simulink model "Factorial_Task"  (R2018b)
settings: Solver=FixedStepDiscrete  StartTime=0.0  StopTime=10.0  RelTol=1e-3
settings Model: Creator=karim  LastModifiedBy=karim
settings OptimizationCC: DefaultParameterBehavior=Inlined  EnhancedBackFolding=on  PassReuseOutputArgsAs=Individual arguments  OptimizeBlockOrder=speed  DifferentSizesBufferReuse=on  OptimizationCustomize=off
settings DebuggingCC: UnderspecifiedInitializationDetection=Classic  MergeDetectMultiDrivingBlocksExec=none  ParameterTunabilityLossMsg=error
settings ModelReferenceCC: PropagateSignalLabelsOutOfModel=off
settings SFSimCC: MATLABDynamicMemAlloc=off
settings RTWCC: SystemTargetFile=ert.tlc  GenCodeOnly=on  TemplateMakefile=ert_default_tmf  GenerateReport=on  IncludeHyperlinkInReport=on  LaunchReport=on  GenerateTraceInfo=on  GenerateTraceReport=on  GenerateTraceReportSl=on  GenerateTraceReportSf=on  GenerateTraceReportEml=on
settings CodeAppCC: ForceParamTrailComments=on  IgnoreCustomStorageClasses=off  OperatorAnnotations=on  SimulinkDataObjDesc=on  SFDataObjDesc=on  InsertBlockDesc=on
settings ERTTargetCC: TargetLangStandard=C99 (ISO)  GenerateSampleERTMain=on  InlinedParameterPlacement=NonHierarchical  ERTCustomFileTemplate=example_file_process.tlc

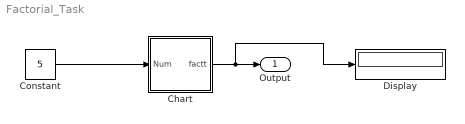
== system Factorial_Task ==
  Chart : Stateflow chart  TreatAsAtomicUnit=on
  Constant : Constant  Value=5  OutDataTypeStr=uint32
  Display : Display
  Output : Outport
  wires:
  Constant/1 -> Chart/1(Num)
  Chart/1(factt) -> Display/1, Output/1

== stateflow chart Factorial_Task/Chart ==
  (default) -> (junction 10) : % Fact
  (junction 11) -> (junction 9) [order 1] : [index<=Num]
  (junction 9) -> (junction 12) : {factt=factt*index;}
  (junction 10) -> (junction 11) : {index=uint32(1);
      | factt=uint32(1);}
  (junction 12) -> (junction 11) : {index=index+1;}
  (junction 11) -> (junction 13) [order 2]
  data: index local uint32; factt output uint32 [0..1000]; Num input uint32 [0..100]
